simulink model "A_Robot_2_0_m_5_V22_SI"  (R2025b)
settings: Solver=VariableStepAuto  StartTime=0.0  StopTime=150  RelTol=1e-3
model workspace (MAT data in the model file):
  Km = [1; 1]
values from neighbouring files (symbols this model uses):
  kcl = kil + 50    (= 75)    [A_init_0.m]    (also in A_init_0_v2.m; A_init_1_v2.m)
  kcr = kir + 50    (= 75)    [A_init_0.m]    (also in A_init_0_v2.m; A_init_1_v2.m)
  kil = 25    [A_init_0.m]    (also in A_init_0_v2.m; A_init_1_v2.m)
  kir = 25    [A_init_0.m]    (also in A_init_0_v2.m; A_init_1_v2.m)
  kpl = 5    [A_init_0.m]    (also in A_init_0_v2.m; A_init_1_v2.m)
  kpr = 5    [A_init_0.m]    (also in A_init_0_v2.m; A_init_1_v2.m)
  theta0 = theta_0_min + (theta_0_max - theta_0_min) * rand()    [A_init_0.m]    (also in A_init_0_v2.m; A_init_1_v2.m)
  theta_gsr = theta_gsr_min + (theta_gsr_max - theta_gsr_min) * rand()    [A_init_0.m]    (also in A_init_0_v2.m; A_init_1_v2.m)
  v_rand = v_rand_0 + (v_rand_max - v_rand_0) * rand()    [A_init_0.m]    (also in A_init_0_v2.m; A_init_1_v2.m)
  x0 = x_0_min + (x_0_max - x_0_min) * rand()    [A_init_0.m]    (also in A_init_0_v2.m; A_init_1_v2.m)
  x_gsr = x_gsr_min + (x_gsr_max - x_gsr_min) * rand()    [A_init_0.m]    (also in A_init_0_v2.m; A_init_1_v2.m)
  y0 = y_0_min + (y_0_max - y_0_min) * rand()    [A_init_0.m]    (also in A_init_0_v2.m; A_init_1_v2.m)
  y_gsr = y_gsr_min + (y_gsr_max - y_gsr_min) * rand()    [A_init_0.m]    (also in A_init_0_v2.m; A_init_1_v2.m)
undefined symbols (not defined in the file or in its folder): DiscIntNeverNeededParam
libraries: simulink x15, rllib x1
(part 2 of 3)

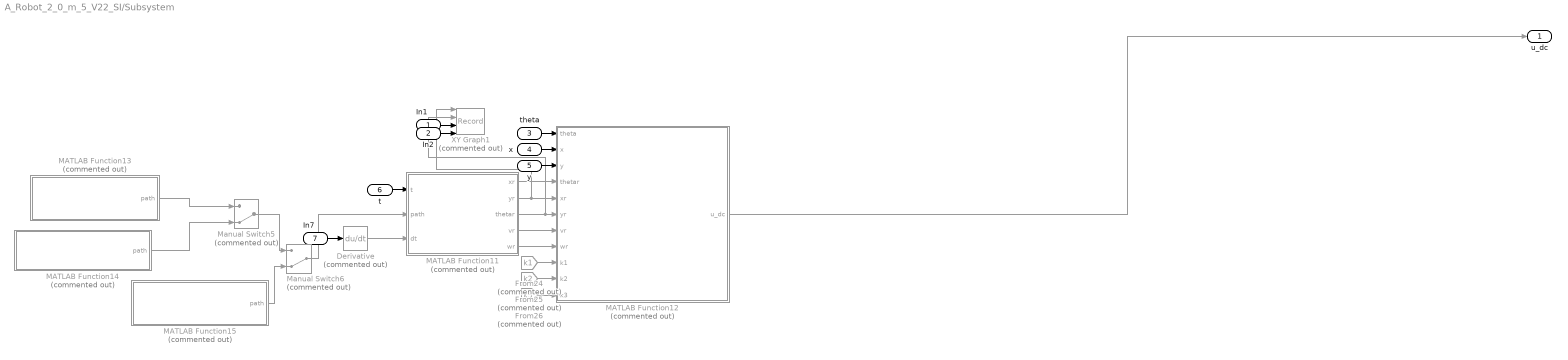
== system A_Robot_2_0_m_5_V22_SI/Subsystem ==
  In1 : Inport
  In2 : Inport  Port=2
  theta : Inport  Port=3
  x : Inport  Port=4
  y : Inport  Port=5
  t : Inport  Port=6
  In7 : Inport  Port=7
  Derivative : Derivative  Commented=on
  From24 : From  Commented=on  GotoTag=k1  TagVisibility=global
  From25 : From  Commented=on  GotoTag=k2  TagVisibility=global
  From26 : From  Commented=on  GotoTag=k3  TagVisibility=global
  MATLAB Function11 : MATLAB Function  Commented=on  TreatAsAtomicUnit=on
  MATLAB Function12 : MATLAB Function  Commented=on  TreatAsAtomicUnit=on
  MATLAB Function13 : MATLAB Function  Commented=on  TreatAsAtomicUnit=on
  MATLAB Function14 : MATLAB Function  Commented=on  TreatAsAtomicUnit=on
  MATLAB Function15 : MATLAB Function  Commented=on  TreatAsAtomicUnit=on
  Manual Switch5 : ManualSwitch  Commented=on  CurrentSetting=0
  Manual Switch6 : ManualSwitch  Commented=on  CurrentSetting=0
  XY Graph1 : Record  Commented=on  NumPorts=4.0  FileSettingsInternal="{\"entries\":[{\"content\":{\"excelSettings\":{\"content\":{},\"type\":\"Streamout.ExcelSettings\"},\"parquetSettings\":{\"content\":{},\"type\":\"Streamout.ParquetSettings\"}},\"type\":\"Streamout.FileSettingStorage\",\"uuid\":\"\"}],\"packageUris\":[\"http:\\/\\/schema.mathworks.com\\/mf0\\/streamout_blocks\\/R2020a\"],\"version\":\"1.0\"}"  FrameSettings=[0, 0, 0, 0]  Layout=[1 1]  SignalsInternal="{\"entries\":[{\"content\":{},\"type\":\"RecordBlkView.InputSignals\",\"uuid\":\"\"}],\"packageUris\":[\"http:\\/\\/schema.mathworks.com\\/mf0\\/streamout_blocks\\/R2020a\"],\"version\":\"1.0\"}"  VisualizationBindings="{\"xyplotplugin\":{\"info\":[{\"series\":[],\"subplotID\":1}]}}"  CompatibilityTag=XY
  u_dc : Outport
  wires:
  Derivative/1 -> MATLAB Function11/3(dt)
  MATLAB Function11/5(wr) -> MATLAB Function12/8(wr)
  MATLAB Function11/1(xr) -> MATLAB Function12/4(thetar)
  Manual Switch5/1 -> Manual Switch6/1
  From26/1 -> MATLAB Function12/11(k3)
  MATLAB Function14/1(path) -> Manual Switch5/2
  Manual Switch6/1 -> MATLAB Function11/2(path)
  MATLAB Function11/3(thetar) -> XY Graph1/2, MATLAB Function12/6(yr)
  MATLAB Function13/1(path) -> Manual Switch5/1
  In2/1 -> XY Graph1/4
  From25/1 -> MATLAB Function12/10(k2)
  MATLAB Function11/2(yr) -> XY Graph1/1, MATLAB Function12/5(xr)
  From24/1 -> MATLAB Function12/9(k1)
  In7/1 -> Derivative/1
  MATLAB Function15/1(path) -> Manual Switch6/2
  MATLAB Function11/4(vr) -> MATLAB Function12/7(vr)
  MATLAB Function12/1(u_dc) -> u_dc/1
  theta/1 -> MATLAB Function12/1(theta)
  x/1 -> MATLAB Function12/2(x)
  y/1 -> MATLAB Function12/3(y)
  t/1 -> MATLAB Function11/1(t)
  In1/1 -> XY Graph1/3

== system A_Robot_2_0_m_5_V22_SI/Subsystem1 ==
  + : Inport
  - : Inport  Port=2
  Demux : Demux  Outputs=2
  Demux4 : Demux  Outputs=2
  Mux7 : Mux  Inputs=2
  Sum5 : Sum  Inputs=-+|
  Sum6 : Sum  Inputs=-+|
  Out : Outport
  wires:
  Demux4/1 -> Sum5/1
  Sum5/1 -> Mux7/1
  Sum6/1 -> Mux7/2
  Demux/2 -> Sum6/2
  Demux4/2 -> Sum6/1
  Mux7/1 -> Out/1
  -/1 -> Demux4/1
  +/1 -> Demux/1
  Demux/1 -> Sum5/2

== system A_Robot_2_0_m_5_V22_SI/Subsystem10 ==
  + : Inport
  - : Inport  Port=2
  Demux : Demux  Outputs=2
  Demux4 : Demux  Outputs=2
  Mux7 : Mux  Inputs=2
  Sum5 : Sum  Inputs=-+|
  Sum6 : Sum  Inputs=-+|
  Out : Outport
  wires:
  Demux4/1 -> Sum5/1
  Sum5/1 -> Mux7/1
  Sum6/1 -> Mux7/2
  Demux/2 -> Sum6/2
  Demux4/2 -> Sum6/1
  Mux7/1 -> Out/1
  -/1 -> Demux4/1
  +/1 -> Demux/1
  Demux/1 -> Sum5/2

== system A_Robot_2_0_m_5_V22_SI/Subsystem2 ==
  + : Inport
  - : Inport  Port=2
  Demux : Demux  Outputs=2
  Demux4 : Demux  Outputs=2
  Mux7 : Mux  Inputs=2
  Sum5 : Sum  Inputs=-+|
  Sum6 : Sum  Inputs=-+|
  Out : Outport
  wires:
  Demux4/1 -> Sum5/1
  Sum5/1 -> Mux7/1
  Sum6/1 -> Mux7/2
  Demux/2 -> Sum6/2
  Demux4/2 -> Sum6/1
  Mux7/1 -> Out/1
  -/1 -> Demux4/1
  +/1 -> Demux/1
  Demux/1 -> Sum5/2

== system A_Robot_2_0_m_5_V22_SI/Subsystem3 ==
  + : Inport
  - : Inport  Port=2
  Demux : Demux  Outputs=3
  Demux4 : Demux  Outputs=3
  Mux7 : Mux  Inputs=3
  Sum1 : Sum  Inputs=-+|
  Sum5 : Sum  Inputs=-+|
  Sum6 : Sum  Inputs=-+|
  Out : Outport
  wires:
  Demux4/1 -> Sum5/1
  Sum5/1 -> Mux7/1
  Sum6/1 -> Mux7/2
  Demux/2 -> Sum6/2
  Demux4/2 -> Sum6/1
  Mux7/1 -> Out/1
  -/1 -> Demux4/1
  +/1 -> Demux/1
  Demux/1 -> Sum5/2
  Demux/3 -> Sum1/2
  Demux4/3 -> Sum1/1
  Sum1/1 -> Mux7/3

== system A_Robot_2_0_m_5_V22_SI/Subsystem4 ==
  + : Inport
  -1 : Inport  Port=2
  Demux : Demux  Outputs=3
  Demux4 : Demux  Outputs=3
  Mux7 : Mux  Inputs=3
  Sum1 : Sum  Inputs=-+|
  Sum5 : Sum  Inputs=-+|
  Sum6 : Sum  Inputs=-+|
  Out : Outport
  wires:
  Demux4/1 -> Sum5/1
  Sum5/1 -> Mux7/1
  Sum6/1 -> Mux7/2
  Demux/2 -> Sum6/2
  Demux4/2 -> Sum6/1
  Mux7/1 -> Out/1
  -1/1 -> Demux4/1
  +/1 -> Demux/1
  Demux/1 -> Sum5/2
  Demux/3 -> Sum1/2
  Demux4/3 -> Sum1/1
  Sum1/1 -> Mux7/3

== system A_Robot_2_0_m_5_V22_SI/Subsystem5 ==
  + : Inport
  - : Inport  Port=2
  Demux : Demux  Outputs=2
  Demux4 : Demux  Outputs=2
  Mux7 : Mux  Inputs=2
  Sum5 : Sum  Inputs=-+|
  Sum6 : Sum  Inputs=-+|
  Out : Outport
  wires:
  Demux4/1 -> Sum5/1
  Sum5/1 -> Mux7/1
  Sum6/1 -> Mux7/2
  Demux/2 -> Sum6/2
  Demux4/2 -> Sum6/1
  Mux7/1 -> Out/1
  -/1 -> Demux4/1
  +/1 -> Demux/1
  Demux/1 -> Sum5/2

== system A_Robot_2_0_m_5_V22_SI/Subsystem6 ==
  + : Inport
  -1 : Inport  Port=2
  Demux : Demux  Outputs=3
  Demux4 : Demux  Outputs=3
  Mux7 : Mux  Inputs=3
  Sum1 : Sum  Inputs=-+|
  Sum5 : Sum  Inputs=-+|
  Sum6 : Sum  Inputs=-+|
  Out : Outport
  wires:
  Demux4/1 -> Sum5/1
  Sum5/1 -> Mux7/1
  Sum6/1 -> Mux7/2
  Demux/2 -> Sum6/2
  Demux4/2 -> Sum6/1
  Mux7/1 -> Out/1
  -1/1 -> Demux4/1
  +/1 -> Demux/1
  Demux/1 -> Sum5/2
  Demux/3 -> Sum1/2
  Demux4/3 -> Sum1/1
  Sum1/1 -> Mux7/3

== system A_Robot_2_0_m_5_V22_SI/Subsystem7 ==
  + : Inport
  - : Inport  Port=2
  Demux : Demux  Outputs=3
  Demux4 : Demux  Outputs=3
  Mux7 : Mux  Inputs=3
  Sum1 : Sum  Inputs=-+|
  Sum5 : Sum  Inputs=-+|
  Sum6 : Sum  Inputs=-+|
  Out : Outport
  wires:
  Demux4/1 -> Sum5/1
  Sum5/1 -> Mux7/1
  Sum6/1 -> Mux7/2
  Demux/2 -> Sum6/2
  Demux4/2 -> Sum6/1
  Mux7/1 -> Out/1
  -/1 -> Demux4/1
  +/1 -> Demux/1
  Demux/1 -> Sum5/2
  Demux/3 -> Sum1/2
  Demux4/3 -> Sum1/1
  Sum1/1 -> Mux7/3

== system A_Robot_2_0_m_5_V22_SI/Subsystem8 ==
  + : Inport
  -1 : Inport  Port=2
  Demux : Demux  Outputs=3
  Demux4 : Demux  Outputs=3
  Mux7 : Mux  Inputs=3
  Sum1 : Sum  Inputs=-+|
  Sum5 : Sum  Inputs=-+|
  Sum6 : Sum  Inputs=-+|
  Out : Outport
  wires:
  Demux4/1 -> Sum5/1
  Sum5/1 -> Mux7/1
  Sum6/1 -> Mux7/2
  Demux/2 -> Sum6/2
  Demux4/2 -> Sum6/1
  Mux7/1 -> Out/1
  -1/1 -> Demux4/1
  +/1 -> Demux/1
  Demux/1 -> Sum5/2
  Demux/3 -> Sum1/2
  Demux4/3 -> Sum1/1
  Sum1/1 -> Mux7/3

== system A_Robot_2_0_m_5_V22_SI/Subsystem9 ==
  + : Inport
  - : Inport  Port=2
  Demux : Demux  Outputs=3
  Demux4 : Demux  Outputs=3
  Mux7 : Mux  Inputs=3
  Sum1 : Sum  Inputs=-+|
  Sum5 : Sum  Inputs=-+|
  Sum6 : Sum  Inputs=-+|
  Out : Outport
  wires:
  Demux4/1 -> Sum5/1
  Sum5/1 -> Mux7/1
  Sum6/1 -> Mux7/2
  Demux/2 -> Sum6/2
  Demux4/2 -> Sum6/1
  Mux7/1 -> Out/1
  -/1 -> Demux4/1
  +/1 -> Demux/1
  Demux/1 -> Sum5/2
  Demux4/3 -> Sum1/1
  Demux/3 -> Sum1/2
  Sum1/1 -> Mux7/3

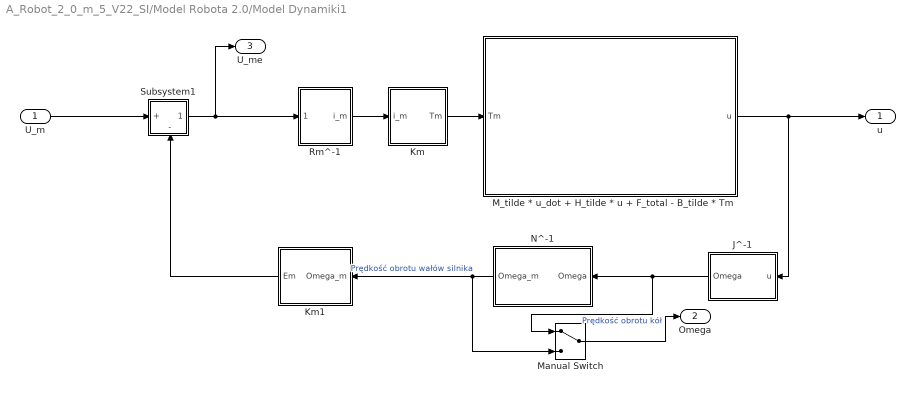
== system A_Robot_2_0_m_5_V22_SI/Model Robota 2.0/Model Dynamiki1 ==
  U_m : Inport
  J^-1 : Subsystem
  Km : Subsystem
  Km1 : Subsystem
  M_tilde * u_dot + H_tilde * u + F_total - B_tilde * Tm : Subsystem
  Manual Switch : ManualSwitch
  N^-1 : Subsystem
  Rm^-1 : Subsystem
  Subsystem1 : Subsystem
      settings: PortSchema="{\"entries\":[{\"content\":{\"sides\":[{\"content\":{\"connectorIds\":[\"In1\"]},\"type\":\"ConnectorPlacement.EquallySpacedRectSide\",\"uuid\":\"f81facd5-8dce-4a5d-a044-cb75bd1df10e\"},{\"content\":{\"connectorIds\":[\"Out1\"],\"side\":\"RIGHT\"},\"type\":\"ConnectorPlacement.EquallySpacedRectSide\",\"uuid\":\"361c4912-9b0e-4ff4-a4c3-0f951cd83b7e\"},{\"content\":{\"side\":\"TOP\"},\"type\":\"ConnectorPlacement.EquallySpacedRectSide\",\"uuid\":\"7c64f9f2-ca51-41c2-8f6b-bbae03c31185\"},{\"content\":{\"connectorIds\":[\"In2\"],\"side\":\"BOTTOM\"},\"type\":\"ConnectorPlacement.EquallySpacedRectSide\",\"uuid\":\"00962904-9a33-4c86-93c6-1e958d83cf78\"}]},\"type\":\"ConnectorPlacement.EquallySpacedConnector\",\"uuid\":\"b3c5fd64-8318-4fc9-b064-dcb9a80ffa17\"}],\"packageUris\":[\"http://schema.mathworks.com/mf0/Connector/R2020b\"],\"version\":\"1.0\"}"
  u : Outport
  Omega : Outport  Port=2
  U_me : Outport  Port=3
  wires:
  M_tilde * u_dot + H_tilde * u + F_total - B_tilde * Tm/1(u) -> J^-1/1(u), u/1
  Rm^-1/1(i_m) -> Km/1(i_m)
  Subsystem1/1(U_me) -> U_me/1, Rm^-1/1(U_me)
  N^-1/1(Omega_m) -> Manual Switch/2, Km1/1(Omega_m)  "Prędkość obrotu wałów silnika"
  J^-1/1(Omega) -> Manual Switch/1, N^-1/1(Omega)  "Prędkość obrotu kół"
  Km1/1(Em) -> Subsystem1/2(-)
  Km/1(Tm) -> M_tilde * u_dot + H_tilde * u + F_total - B_tilde * Tm/1(Tm)
  U_m/1 -> Subsystem1/1(+)
  Manual Switch/1 -> Omega/1

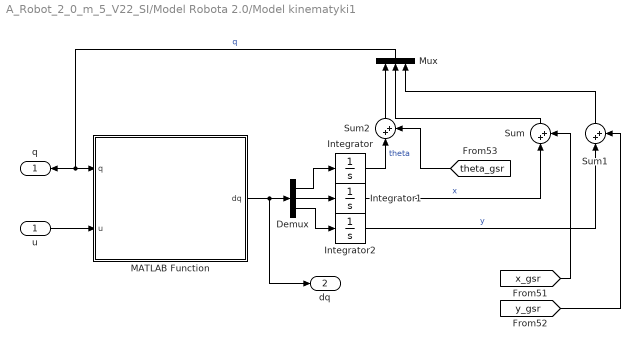
== system A_Robot_2_0_m_5_V22_SI/Model Robota 2.0/Model kinematyki1 ==
  u : Inport
  Demux : Demux  Outputs=3
  Integrator : Integrator
  Integrator1 : Integrator
  Integrator2 : Integrator
  MATLAB Function : MATLAB Function  TreatAsAtomicUnit=on
  Mux : Mux  Inputs=3
  Sum : Sum  Inputs=|++
  Sum1 : Sum  Inputs=|++
  Sum2 : Sum  Inputs=|++
  q : Outport
  dq : Outport  Port=2
  wires:
  Mux/1 -> q/1, MATLAB Function/1(q)  "q"
  Demux/1 -> Integrator/1
  Demux/3 -> Integrator2/1
  Demux/2 -> Integrator1/1
  Integrator2/1 -> Sum1/1  "y"
  MATLAB Function/1(dq) -> dq/1, Demux/1
  Integrator/1 -> Sum2/1  "theta"
  Integrator1/1 -> Sum/1  "x"
  u/1 -> MATLAB Function/2(u)
  [y_gsr] -> Sum1/2
  [x_gsr] -> Sum/2
  Sum/1 -> Mux/2
  Sum1/1 -> Mux/3
  [theta_gsr] -> Sum2/2
  Sum2/1 -> Mux/1

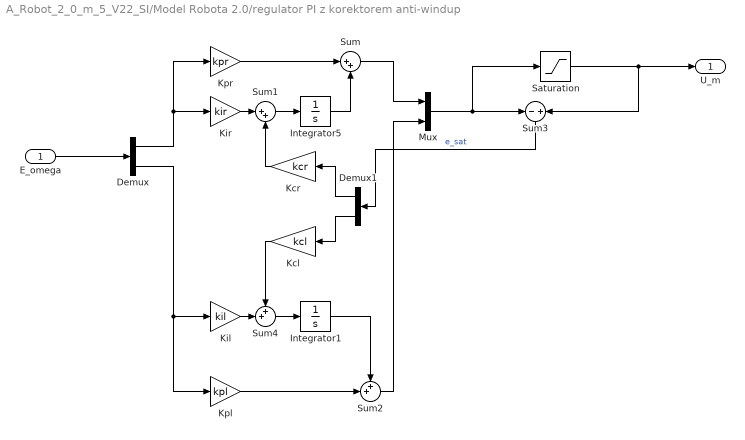
== system A_Robot_2_0_m_5_V22_SI/Model Robota 2.0/regulator PI z korektorem anti-windup ==
  E_omega : Inport
  Demux : Demux  Outputs=2
  Demux1 : Demux  Outputs=2
  Integrator1 : Integrator
  Integrator5 : Integrator
  Kcl : Gain  Gain=kcl
  Kcr : Gain  Gain=kcr
  Kil : Gain  Gain=kil
  Kir : Gain  Gain=kir
  Kpl : Gain  Gain=kpl
  Kpr : Gain  Gain=kpr
  Mux : Mux  Inputs=2
  Saturation : Saturate  UpperLimit=12  LowerLimit=-12
  Sum : Sum  Inputs=|++
  Sum1 : Sum  Inputs=|++
  Sum2 : Sum  Inputs=++|
  Sum3 : Sum  Inputs=-|+
  Sum4 : Sum  Inputs=++|
  U_m : Outport
  wires:
  Kcr/1 -> Sum1/2
  Kpr/1 -> Sum/1
  Integrator5/1 -> Sum/2
  Kir/1 -> Sum1/1
  Sum1/1 -> Integrator5/1
  Saturation/1 -> Sum3/2, U_m/1
  E_omega/1 -> Demux/1
  Demux/1 -> Kir/1, Kpr/1
  Kcl/1 -> Sum4/1
  Sum4/1 -> Integrator1/1
  Kpl/1 -> Sum2/2
  Integrator1/1 -> Sum2/1
  Kil/1 -> Sum4/2
  Demux/2 -> Kil/1, Kpl/1
  Sum3/1 -> Demux1/1  "e_sat"
  Demux1/1 -> Kcr/1
  Demux1/2 -> Kcl/1
  Sum/1 -> Mux/1
  Sum2/1 -> Mux/2
  Mux/1 -> Saturation/1, Sum3/1

== system A_Robot_2_0_m_5_V22_SI/Model Robota 2.1/Model Dynamiki1 ==
  U_m : Inport
  J^-1 : Subsystem
  Km : Subsystem
  Km1 : Subsystem
  M_tilde * u_dot + H_tilde * u + F_total - B_tilde * Tm : Subsystem
  Manual Switch : ManualSwitch
  N^-1 : Subsystem
  Rm^-1 : Subsystem
  Subsystem1 : Subsystem
      settings: PortSchema="{\"entries\":[{\"content\":{\"sides\":[{\"content\":{\"connectorIds\":[\"In1\"]},\"type\":\"ConnectorPlacement.EquallySpacedRectSide\",\"uuid\":\"f81facd5-8dce-4a5d-a044-cb75bd1df10e\"},{\"content\":{\"connectorIds\":[\"Out1\"],\"side\":\"RIGHT\"},\"type\":\"ConnectorPlacement.EquallySpacedRectSide\",\"uuid\":\"361c4912-9b0e-4ff4-a4c3-0f951cd83b7e\"},{\"content\":{\"side\":\"TOP\"},\"type\":\"ConnectorPlacement.EquallySpacedRectSide\",\"uuid\":\"7c64f9f2-ca51-41c2-8f6b-bbae03c31185\"},{\"content\":{\"connectorIds\":[\"In2\"],\"side\":\"BOTTOM\"},\"type\":\"ConnectorPlacement.EquallySpacedRectSide\",\"uuid\":\"00962904-9a33-4c86-93c6-1e958d83cf78\"}]},\"type\":\"ConnectorPlacement.EquallySpacedConnector\",\"uuid\":\"b3c5fd64-8318-4fc9-b064-dcb9a80ffa17\"}],\"packageUris\":[\"http://schema.mathworks.com/mf0/Connector/R2020b\"],\"version\":\"1.0\"}"
  u : Outport
  Omega : Outport  Port=2
  U_me : Outport  Port=3
  wires:
  M_tilde * u_dot + H_tilde * u + F_total - B_tilde * Tm/1(u) -> J^-1/1(u), u/1
  Rm^-1/1(i_m) -> Km/1(i_m)
  Subsystem1/1(U_me) -> U_me/1, Rm^-1/1(U_me)
  N^-1/1(Omega_m) -> Manual Switch/2, Km1/1(Omega_m)  "Prędkość obrotu wałów silnika"
  J^-1/1(Omega) -> Manual Switch/1, N^-1/1(Omega)  "Prędkość obrotu kół"
  Km1/1(Em) -> Subsystem1/2(-)
  Km/1(Tm) -> M_tilde * u_dot + H_tilde * u + F_total - B_tilde * Tm/1(Tm)
  U_m/1 -> Subsystem1/1(+)
  Manual Switch/1 -> Omega/1

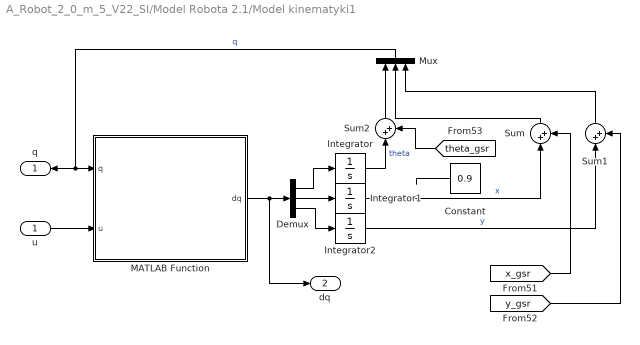
== system A_Robot_2_0_m_5_V22_SI/Model Robota 2.1/Model kinematyki1 ==
  u : Inport
  Constant : Constant  Value=0.9
  Demux : Demux  Outputs=3
  Integrator : Integrator
  Integrator1 : Integrator
  Integrator2 : Integrator
  MATLAB Function : MATLAB Function  TreatAsAtomicUnit=on
  Mux : Mux  Inputs=3
  Sum : Sum  Inputs=|++
  Sum1 : Sum  Inputs=|++
  Sum2 : Sum  Inputs=|++
  q : Outport
  dq : Outport  Port=2
  wires:
  Mux/1 -> q/1, MATLAB Function/1(q)  "q"
  Demux/1 -> Integrator/1
  Demux/3 -> Integrator2/1
  Demux/2 -> Integrator1/1
  Integrator2/1 -> Sum1/1  "y"
  MATLAB Function/1(dq) -> dq/1, Demux/1
  Integrator/1 -> Sum2/1  "theta"
  Integrator1/1 -> Sum/1  "x"
  u/1 -> MATLAB Function/2(u)
  [y_gsr] -> Sum1/2
  [x_gsr] -> Sum/2
  Sum/1 -> Mux/2
  Sum1/1 -> Mux/3
  [theta_gsr] -> Sum2/2
  Sum2/1 -> Mux/1
  Constant/1 -> ?

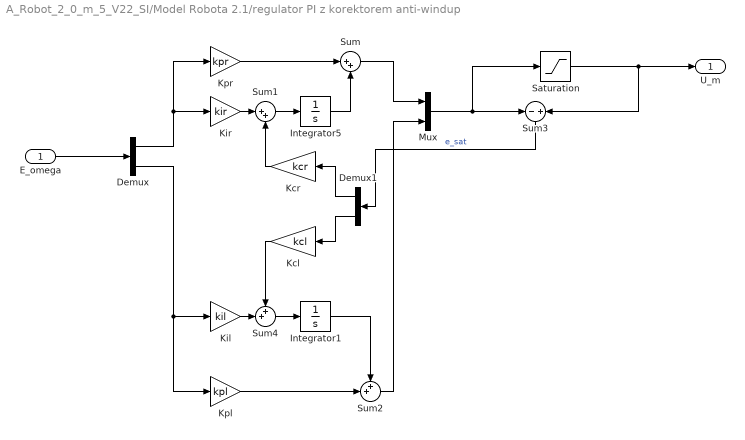
== system A_Robot_2_0_m_5_V22_SI/Model Robota 2.1/regulator PI z korektorem anti-windup ==
  E_omega : Inport
  Demux : Demux  Outputs=2
  Demux1 : Demux  Outputs=2
  Integrator1 : Integrator
  Integrator5 : Integrator
  Kcl : Gain  Gain=kcl
  Kcr : Gain  Gain=kcr
  Kil : Gain  Gain=kil
  Kir : Gain  Gain=kir
  Kpl : Gain  Gain=kpl
  Kpr : Gain  Gain=kpr
  Mux : Mux  Inputs=2
  Saturation : Saturate  UpperLimit=12  LowerLimit=-12
  Sum : Sum  Inputs=|++
  Sum1 : Sum  Inputs=|++
  Sum2 : Sum  Inputs=++|
  Sum3 : Sum  Inputs=-|+
  Sum4 : Sum  Inputs=++|
  U_m : Outport
  wires:
  Kcr/1 -> Sum1/2
  Kpr/1 -> Sum/1
  Integrator5/1 -> Sum/2
  Kir/1 -> Sum1/1
  Sum1/1 -> Integrator5/1
  Saturation/1 -> Sum3/2, U_m/1
  E_omega/1 -> Demux/1
  Demux/1 -> Kir/1, Kpr/1
  Kcl/1 -> Sum4/1
  Sum4/1 -> Integrator1/1
  Kpl/1 -> Sum2/2
  Integrator1/1 -> Sum2/1
  Kil/1 -> Sum4/2
  Demux/2 -> Kil/1, Kpl/1
  Sum3/1 -> Demux1/1  "e_sat"
  Demux1/1 -> Kcr/1
  Demux1/2 -> Kcl/1
  Sum/1 -> Mux/1
  Sum2/1 -> Mux/2
  Mux/1 -> Saturation/1, Sum3/1

== system A_Robot_2_0_m_5_V22_SI/Nagroda/Subsystem ==
  In1 : Inport
  Sqrt : Sqrt
  Square : Math  Operator=square
  Out1 : Outport
  wires:
  Square/1 -> Sqrt/1
  In1/1 -> Square/1
  Sqrt/1 -> Out1/1

== system A_Robot_2_0_m_5_V22_SI/Nagroda/Subsystem1 ==
  In1 : Inport
  Sqrt : Sqrt
  Square : Math  Operator=square
  Out1 : Outport
  wires:
  Square/1 -> Sqrt/1
  In1/1 -> Square/1
  Sqrt/1 -> Out1/1

== system A_Robot_2_0_m_5_V22_SI/Nagroda/Subsystem2 ==
  In1 : Inport
  Sqrt : Sqrt
  Square : Math  Operator=square
  Out1 : Outport
  wires:
  Square/1 -> Sqrt/1
  In1/1 -> Square/1
  Sqrt/1 -> Out1/1

== system A_Robot_2_0_m_5_V22_SI/Nagroda/Subsystem3 ==
  In1 : Inport
  Sqrt : Sqrt
  Square : Math  Operator=square
  Out1 : Outport
  wires:
  Square/1 -> Sqrt/1
  In1/1 -> Square/1
  Sqrt/1 -> Out1/1

== system A_Robot_2_0_m_5_V22_SI/Nagroda/Subsystem4 ==
  In1 : Inport
  Sqrt : Sqrt
  Square : Math  Operator=square
  Out1 : Outport
  wires:
  Square/1 -> Sqrt/1
  In1/1 -> Square/1
  Sqrt/1 -> Out1/1

== system A_Robot_2_0_m_5_V22_SI/Nagroda/Subsystem5 ==
  In1 : Inport
  Sqrt : Sqrt
  Square : Math  Operator=square
  Out1 : Outport
  wires:
  Square/1 -> Sqrt/1
  In1/1 -> Square/1
  Sqrt/1 -> Out1/1

== system A_Robot_2_0_m_5_V22_SI/Nagroda/Subsystem6 ==
  In1 : Inport
  Sqrt : Sqrt
  Square : Math  Operator=square
  Out1 : Outport
  wires:
  Square/1 -> Sqrt/1
  In1/1 -> Square/1
  Sqrt/1 -> Out1/1

== system A_Robot_2_0_m_5_V22_SI/Nagroda/Subsystem7 ==
  In1 : Inport
  Sqrt : Sqrt
  Square : Math  Operator=square
  Out1 : Outport
  wires:
  Square/1 -> Sqrt/1
  In1/1 -> Square/1
  Sqrt/1 -> Out1/1

== system A_Robot_2_0_m_5_V22_SI/Model Robota 2.0/Model Dynamiki1/J^-1 ==
  u : Inport
  MATLAB Function2 : MATLAB Function  TreatAsAtomicUnit=on
  Omega : Outport
  wires:
  MATLAB Function2/1(Omega) -> Omega/1
  [r] -> MATLAB Function2/3(r)
  [b] -> MATLAB Function2/2(b)
  u/1 -> MATLAB Function2/1(u)

== system A_Robot_2_0_m_5_V22_SI/Model Robota 2.0/Model Dynamiki1/Km ==
  i_m : Inport
  MATLAB Function2 : MATLAB Function  TreatAsAtomicUnit=on
  Tm : Outport
  wires:
  [Km] -> MATLAB Function2/2(km)
  i_m/1 -> MATLAB Function2/1(i_m)
  MATLAB Function2/1(Tm) -> Tm/1

== system A_Robot_2_0_m_5_V22_SI/Model Robota 2.0/Model Dynamiki1/Km1 ==
  Omega_m : Inport
  MATLAB Function2 : MATLAB Function  TreatAsAtomicUnit=on
  Em : Outport
  wires:
  [Km] -> MATLAB Function2/2(km)
  Omega_m/1 -> MATLAB Function2/1(Omega_m)
  MATLAB Function2/1(Em) -> Em/1

== system A_Robot_2_0_m_5_V22_SI/Model Robota 2.0/Model Dynamiki1/M_tilde * u_dot + H_tilde * u + F_total - B_tilde * Tm ==
  Tm : Inport
  B~ : Subsystem
  Demux : Demux  Outputs=2
  Fa(u) + Fr : Subsystem
  H~ : Subsystem
  Integrator : Integrator
  Integrator1 : Integrator
  Mux : Mux  Inputs=2
  M~ : Subsystem
  Subsystem1 : Subsystem
      settings: PortSchema="{\"entries\":[{\"content\":{\"sides\":[{\"content\":{\"connectorIds\":[\"In1\"]},\"type\":\"ConnectorPlacement.EquallySpacedRectSide\",\"uuid\":\"f81facd5-8dce-4a5d-a044-cb75bd1df10e\"},{\"content\":{\"connectorIds\":[\"Out1\"],\"side\":\"RIGHT\"},\"type\":\"ConnectorPlacement.EquallySpacedRectSide\",\"uuid\":\"361c4912-9b0e-4ff4-a4c3-0f951cd83b7e\"},{\"content\":{\"connectorIds\":[\"In2\"],\"side\":\"TOP\"},\"type\":\"ConnectorPlacement.EquallySpacedRectSide\",\"uuid\":\"7c64f9f2-ca51-41c2-8f6b-bbae03c31185\"},{\"content\":{\"connectorIds\":[\"In3\"],\"side\":\"BOTTOM\"},\"type\":\"ConnectorPlacement.EquallySpacedRectSide\",\"uuid\":\"00962904-9a33-4c86-93c6-1e958d83cf78\"}]},\"type\":\"ConnectorPlacement.EquallySpacedConnector\",\"uuid\":\"b3c5fd64-8318-4fc9-b064-dcb9a80ffa17\"}],\"packageUris\":[\"http://schema.mathworks.com/mf0/Connector/R2020b\"],\"version\":\"1.0\"}"
  u : Outport
  wires:
  Fa(u) + Fr/1(OUT) -> Subsystem1/2(-)
  Mux/1 -> u/1, H~/1(u), Fa(u) + Fr/1(u)  "u"
  Subsystem1/1(Out) -> M~/1(BTm)
  H~/1(OUTH) -> Subsystem1/3(-1)
  M~/1(u_d) -> Demux/1
  B~/1(BTm) -> Subsystem1/1(+)
  Tm/1 -> B~/1(Tm)
  Demux/1 -> Integrator/1
  Integrator/1 -> Mux/1
  Demux/2 -> Integrator1/1
  Integrator1/1 -> Mux/2

== system A_Robot_2_0_m_5_V22_SI/Model Robota 2.0/Model Dynamiki1/N^-1 ==
  Omega : Inport
  MATLAB Function2 : MATLAB Function  TreatAsAtomicUnit=on
  Omega_m : Outport
  wires:
  [ng] -> MATLAB Function2/2(ng)
  Omega/1 -> MATLAB Function2/1(Omega)
  MATLAB Function2/1(Omega_m) -> Omega_m/1

== system A_Robot_2_0_m_5_V22_SI/Model Robota 2.0/Model Dynamiki1/Rm^-1 ==
  U_me : Inport
  MATLAB Function : MATLAB Function  TreatAsAtomicUnit=on
  i_m : Outport
  wires:
  [R] -> MATLAB Function/2(R)
  U_me/1 -> MATLAB Function/1(U_me)
  MATLAB Function/1(i_m) -> i_m/1

== system A_Robot_2_0_m_5_V22_SI/Model Robota 2.0/Model Dynamiki1/Subsystem1 ==
  + : Inport
  - : Inport  Port=2
  Demux : Demux  Outputs=2
  Demux4 : Demux  Outputs=2
  Mux7 : Mux  Inputs=2
  Sum5 : Sum  Inputs=-+|
  Sum6 : Sum  Inputs=-+|
  U_me : Outport
  wires:
  Demux4/1 -> Sum5/1
  Sum5/1 -> Mux7/1
  Sum6/1 -> Mux7/2
  Demux/2 -> Sum6/2
  Demux4/2 -> Sum6/1
  Mux7/1 -> U_me/1
  -/1 -> Demux4/1
  +/1 -> Demux/1
  Demux/1 -> Sum5/2

== system A_Robot_2_0_m_5_V22_SI/Model Robota 2.1/Model Dynamiki1/J^-1 ==
  u : Inport
  MATLAB Function2 : MATLAB Function  TreatAsAtomicUnit=on
  Omega : Outport
  wires:
  MATLAB Function2/1(Omega) -> Omega/1
  [r] -> MATLAB Function2/3(r)
  [b] -> MATLAB Function2/2(b)
  u/1 -> MATLAB Function2/1(u)

== system A_Robot_2_0_m_5_V22_SI/Model Robota 2.1/Model Dynamiki1/Km ==
  i_m : Inport
  MATLAB Function2 : MATLAB Function  TreatAsAtomicUnit=on
  Tm : Outport
  wires:
  [Km] -> MATLAB Function2/2(km)
  i_m/1 -> MATLAB Function2/1(i_m)
  MATLAB Function2/1(Tm) -> Tm/1

== system A_Robot_2_0_m_5_V22_SI/Model Robota 2.1/Model Dynamiki1/Km1 ==
  Omega_m : Inport
  MATLAB Function2 : MATLAB Function  TreatAsAtomicUnit=on
  Em : Outport
  wires:
  [Km] -> MATLAB Function2/2(km)
  Omega_m/1 -> MATLAB Function2/1(Omega_m)
  MATLAB Function2/1(Em) -> Em/1

== system A_Robot_2_0_m_5_V22_SI/Model Robota 2.1/Model Dynamiki1/M_tilde * u_dot + H_tilde * u + F_total - B_tilde * Tm ==
  Tm : Inport
  B~ : Subsystem
  Demux : Demux  Outputs=2
  Fa(u) + Fr : Subsystem
  H~ : Subsystem
  Integrator : Integrator
  Integrator1 : Integrator
  Mux : Mux  Inputs=2
  M~ : Subsystem
  Subsystem1 : Subsystem
      settings: PortSchema="{\"entries\":[{\"content\":{\"sides\":[{\"content\":{\"connectorIds\":[\"In1\"]},\"type\":\"ConnectorPlacement.EquallySpacedRectSide\",\"uuid\":\"f81facd5-8dce-4a5d-a044-cb75bd1df10e\"},{\"content\":{\"connectorIds\":[\"Out1\"],\"side\":\"RIGHT\"},\"type\":\"ConnectorPlacement.EquallySpacedRectSide\",\"uuid\":\"361c4912-9b0e-4ff4-a4c3-0f951cd83b7e\"},{\"content\":{\"connectorIds\":[\"In2\"],\"side\":\"TOP\"},\"type\":\"ConnectorPlacement.EquallySpacedRectSide\",\"uuid\":\"7c64f9f2-ca51-41c2-8f6b-bbae03c31185\"},{\"content\":{\"connectorIds\":[\"In3\"],\"side\":\"BOTTOM\"},\"type\":\"ConnectorPlacement.EquallySpacedRectSide\",\"uuid\":\"00962904-9a33-4c86-93c6-1e958d83cf78\"}]},\"type\":\"ConnectorPlacement.EquallySpacedConnector\",\"uuid\":\"b3c5fd64-8318-4fc9-b064-dcb9a80ffa17\"}],\"packageUris\":[\"http://schema.mathworks.com/mf0/Connector/R2020b\"],\"version\":\"1.0\"}"
  u : Outport
  wires:
  Fa(u) + Fr/1(OUT) -> Subsystem1/2(-)
  Mux/1 -> u/1, H~/1(u), Fa(u) + Fr/1(u)  "u"
  Subsystem1/1(Out) -> M~/1(BTm)
  H~/1(OUTH) -> Subsystem1/3(-1)
  M~/1(u_d) -> Demux/1
  B~/1(BTm) -> Subsystem1/1(+)
  Tm/1 -> B~/1(Tm)
  Demux/1 -> Integrator/1
  Integrator/1 -> Mux/1
  Demux/2 -> Integrator1/1
  Integrator1/1 -> Mux/2

== system A_Robot_2_0_m_5_V22_SI/Model Robota 2.1/Model Dynamiki1/N^-1 ==
  Omega : Inport
  MATLAB Function2 : MATLAB Function  TreatAsAtomicUnit=on
  Omega_m : Outport
  wires:
  [ng] -> MATLAB Function2/2(ng)
  Omega/1 -> MATLAB Function2/1(Omega)
  MATLAB Function2/1(Omega_m) -> Omega_m/1

== system A_Robot_2_0_m_5_V22_SI/Model Robota 2.1/Model Dynamiki1/Rm^-1 ==
  U_me : Inport
  MATLAB Function : MATLAB Function  TreatAsAtomicUnit=on
  i_m : Outport
  wires:
  [R] -> MATLAB Function/2(R)
  U_me/1 -> MATLAB Function/1(U_me)
  MATLAB Function/1(i_m) -> i_m/1

== system A_Robot_2_0_m_5_V22_SI/Model Robota 2.1/Model Dynamiki1/Subsystem1 ==
  + : Inport
  - : Inport  Port=2
  Demux : Demux  Outputs=2
  Demux4 : Demux  Outputs=2
  Mux7 : Mux  Inputs=2
  Sum5 : Sum  Inputs=-+|
  Sum6 : Sum  Inputs=-+|
  U_me : Outport
  wires:
  Demux4/1 -> Sum5/1
  Sum5/1 -> Mux7/1
  Sum6/1 -> Mux7/2
  Demux/2 -> Sum6/2
  Demux4/2 -> Sum6/1
  Mux7/1 -> U_me/1
  -/1 -> Demux4/1
  +/1 -> Demux/1
  Demux/1 -> Sum5/2

== system A_Robot_2_0_m_5_V22_SI/Model Robota 2.0/Model Dynamiki1/M_tilde * u_dot + H_tilde * u + F_total - B_tilde * Tm/B~ ==
  Tm : Inport
  MATLAB Function8 : MATLAB Function  TreatAsAtomicUnit=on
  BTm : Outport
  wires:
  [b] -> MATLAB Function8/2(b)
  [r] -> MATLAB Function8/3(r)
  [ng] -> MATLAB Function8/4(ng)
  MATLAB Function8/1(BTm) -> BTm/1
  Tm/1 -> MATLAB Function8/1(Tm)

== system A_Robot_2_0_m_5_V22_SI/Model Robota 2.0/Model Dynamiki1/M_tilde * u_dot + H_tilde * u + F_total - B_tilde * Tm/Fa(u) + Fr ==
  u : Inport
  Demux : Demux  Outputs=2
  MATLAB Function7 : MATLAB Function  TreatAsAtomicUnit=on
  OUT : Outport
  wires:
  u/1 -> Demux/1
  [r] -> MATLAB Function7/3(r)
  [m] -> MATLAB Function7/4(m)
  [b] -> MATLAB Function7/5(b)
  MATLAB Function7/1(OUT) -> OUT/1
  Demux/1 -> MATLAB Function7/1(omega)
  Demux/2 -> MATLAB Function7/2(v)

== system A_Robot_2_0_m_5_V22_SI/Model Robota 2.0/Model Dynamiki1/M_tilde * u_dot + H_tilde * u + F_total - B_tilde * Tm/H~ ==
  u : Inport
  MATLAB Function6 : MATLAB Function  TreatAsAtomicUnit=on
  OUTH : Outport
  wires:
  [r] -> MATLAB Function6/5(r)
  [b] -> MATLAB Function6/6(b)
  [xi_m] -> MATLAB Function6/3(xi_m)
  MATLAB Function6/1(OUTH) -> OUTH/1
  [xi] -> MATLAB Function6/2(xi)
  [ng] -> MATLAB Function6/4(ng)
  u/1 -> MATLAB Function6/1(u)

== system A_Robot_2_0_m_5_V22_SI/Model Robota 2.0/Model Dynamiki1/M_tilde * u_dot + H_tilde * u + F_total - B_tilde * Tm/M~ ==
  BTm : Inport
  MATLAB Function : MATLAB Function  TreatAsAtomicUnit=on
  MATLAB Function2 : MATLAB Function  TreatAsAtomicUnit=on
  u_d : Outport
  wires:
  [r] -> MATLAB Function/6(r)
  [In] -> MATLAB Function/4(Im)
  [m] -> MATLAB Function2/1(m)
  [m] -> MATLAB Function/5(m)
  [b] -> MATLAB Function/7(b)
  MATLAB Function2/1(Ic) -> MATLAB Function/2(Ic)
  [ng] -> MATLAB Function/8(ng)
  [b] -> MATLAB Function2/2(b)
  [Ik] -> MATLAB Function/3(Ik)
  BTm/1 -> MATLAB Function/1(BTm)
  MATLAB Function/1(u_d) -> u_d/1

== system A_Robot_2_0_m_5_V22_SI/Model Robota 2.0/Model Dynamiki1/M_tilde * u_dot + H_tilde * u + F_total - B_tilde * Tm/Subsystem1 ==
  + : Inport
  - : Inport  Port=2
  -1 : Inport  Port=3
  Demux : Demux  Outputs=2
  Demux1 : Demux  Outputs=2
  Demux4 : Demux  Outputs=2
  Mux7 : Mux  Inputs=2
  Sum1 : Sum  Inputs=-+-|
  Sum5 : Sum  Inputs=-+-|
  Out : Outport
  wires:
  Demux4/1 -> Sum5/1
  Sum5/1 -> Mux7/1
  Sum1/1 -> Mux7/2
  Demux/2 -> Sum1/2
  Demux4/2 -> Sum1/1
  Mux7/1 -> Out/1
  -/1 -> Demux4/1
  +/1 -> Demux/1
  Demux/1 -> Sum5/2
  -1/1 -> Demux1/1
  Demux1/1 -> Sum5/3
  Demux1/2 -> Sum1/3

== system A_Robot_2_0_m_5_V22_SI/Model Robota 2.1/Model Dynamiki1/M_tilde * u_dot + H_tilde * u + F_total - B_tilde * Tm/B~ ==
  Tm : Inport
  MATLAB Function8 : MATLAB Function  TreatAsAtomicUnit=on
  BTm : Outport
  wires:
  [b] -> MATLAB Function8/2(b)
  [r] -> MATLAB Function8/3(r)
  [ng] -> MATLAB Function8/4(ng)
  MATLAB Function8/1(BTm) -> BTm/1
  Tm/1 -> MATLAB Function8/1(Tm)

== system A_Robot_2_0_m_5_V22_SI/Model Robota 2.1/Model Dynamiki1/M_tilde * u_dot + H_tilde * u + F_total - B_tilde * Tm/Fa(u) + Fr ==
  u : Inport
  Demux : Demux  Outputs=2
  MATLAB Function7 : MATLAB Function  TreatAsAtomicUnit=on
  OUT : Outport
  wires:
  u/1 -> Demux/1
  [r] -> MATLAB Function7/3(r)
  [m] -> MATLAB Function7/4(m)
  [b] -> MATLAB Function7/5(b)
  MATLAB Function7/1(OUT) -> OUT/1
  Demux/1 -> MATLAB Function7/1(omega)
  Demux/2 -> MATLAB Function7/2(v)

== system A_Robot_2_0_m_5_V22_SI/Model Robota 2.1/Model Dynamiki1/M_tilde * u_dot + H_tilde * u + F_total - B_tilde * Tm/H~ ==
  u : Inport
  MATLAB Function6 : MATLAB Function  TreatAsAtomicUnit=on
  OUTH : Outport
  wires:
  [r] -> MATLAB Function6/5(r)
  [b] -> MATLAB Function6/6(b)
  [xi_m] -> MATLAB Function6/3(xi_m)
  MATLAB Function6/1(OUTH) -> OUTH/1
  [xi] -> MATLAB Function6/2(xi)
  [ng] -> MATLAB Function6/4(ng)
  u/1 -> MATLAB Function6/1(u)

== system A_Robot_2_0_m_5_V22_SI/Model Robota 2.1/Model Dynamiki1/M_tilde * u_dot + H_tilde * u + F_total - B_tilde * Tm/M~ ==
  BTm : Inport
  MATLAB Function : MATLAB Function  TreatAsAtomicUnit=on
  MATLAB Function2 : MATLAB Function  TreatAsAtomicUnit=on
  u_d : Outport
  wires:
  [r] -> MATLAB Function/6(r)
  [In] -> MATLAB Function/4(Im)
  [m] -> MATLAB Function2/1(m)
  [m] -> MATLAB Function/5(m)
  [b] -> MATLAB Function/7(b)
  MATLAB Function2/1(Ic) -> MATLAB Function/2(Ic)
  [ng] -> MATLAB Function/8(ng)
  [b] -> MATLAB Function2/2(b)
  [Ik] -> MATLAB Function/3(Ik)
  BTm/1 -> MATLAB Function/1(BTm)
  MATLAB Function/1(u_d) -> u_d/1

== system A_Robot_2_0_m_5_V22_SI/Model Robota 2.1/Model Dynamiki1/M_tilde * u_dot + H_tilde * u + F_total - B_tilde * Tm/Subsystem1 ==
  + : Inport
  - : Inport  Port=2
  -1 : Inport  Port=3
  Demux : Demux  Outputs=2
  Demux1 : Demux  Outputs=2
  Demux4 : Demux  Outputs=2
  Mux7 : Mux  Inputs=2
  Sum1 : Sum  Inputs=-+-|
  Sum5 : Sum  Inputs=-+-|
  Out : Outport
  wires:
  Demux4/1 -> Sum5/1
  Sum5/1 -> Mux7/1
  Sum1/1 -> Mux7/2
  Demux/2 -> Sum1/2
  Demux4/2 -> Sum1/1
  Mux7/1 -> Out/1
  -/1 -> Demux4/1
  +/1 -> Demux/1
  Demux/1 -> Sum5/2
  -1/1 -> Demux1/1
  Demux1/1 -> Sum5/3
  Demux1/2 -> Sum1/3

== matlab function A_Robot_2_0_m_5_V22_SI/J^-1/MATLAB Function8 ==
  data: u_dc input; Omega_dc output; r input; b input
function Omega_dc  = konwersja(u_dc, r, b)
    % Przekształcenie prędkości platformy na prędkości kół
    
    
    % Macierz J^{-1} przekształcająca u -> Omega
J_1 = [b/r, 1/r;
      -b/r, 1/r];
    % Obliczenie prędkości kątowych kół
    Omega_dc = J_1 * u_dc;


end

== matlab function A_Robot_2_0_m_5_V22_SI/MATLAB Function9 ==
  data: v_rand input; t input; theta_d_out output; dx_d output; dy_d output; theta_d input; v_d output
function [theta_d_out, dx_d, dy_d, v_d] = GSR(v_rand, t, theta_d)
    v_d = v_rand;
    dx_d = v_d * cos(theta_d);
    dy_d = v_d * sin(theta_d);
    theta_d_out = theta_d;

end

== matlab function A_Robot_2_0_m_5_V22_SI/MATLAB Function10 ==
  data: t input; dtheta_d output
function dtheta_d = obl_theta(t)
    omega_d =0.0;
    dtheta_d = omega_d;

end

== matlab function A_Robot_2_0_m_5_V22_SI/Subsystem/MATLAB Function11 ==
  data: t input; xr output; path input; dt input; yr output; thetar output; vr output; wr output
function [xr, yr, thetar, vr, wr] = GSR_from_path(t, path, dt)
    % Generator sygnałów referencyjnych ze ścieżki (dowolnego wykresu)
    % path: Nx2 macierz punktów [x y]
    % t: czas
    % dt: krok czasowy symulacji

    % Przejście po punktach w tempie odpowiadającym dt
    i = floor(t / dt) + 1;
    i_next = min(i + 1, size(path, 1));
    
    % Bieżący i kolejny punkt
    p1 = path(i, :);
    p2 = path(i_next, :);

    % Pozycja referencyjna
    xr = p1(1);
    yr = p1(2);

    % Różnice
    dx = p2(1) - p1(1);
    dy = p2(2) - p1(2);

    % Prędkość liniowa (różniczkowanie)
    vr = sqrt(dx^2 + dy^2) / dt;

    % Orientacja (kierunek trajektorii)
    thetar = atan2(dy, dx);

    % Przybliżona prędkość kątowa (zmiana kierunku)
    if i < size(path, 1) - 1
        p3 = path(min(i + 2, size(path, 1)), :);
        dtheta1 = atan2(p2(2) - p1(2), p2(1) - p1(1));
        dtheta2 = atan2(p3(2) - p2(2), p3(1) - p2(1));
        dtheta = wrapToPi(dtheta2 - dtheta1);
        wr = dtheta / dt;
    else
        wr = 0;
    end
end

== matlab function A_Robot_2_0_m_5_V22_SI/Subsystem/MATLAB Function12 ==
  data: theta input; x input; y input; thetar input; xr input; yr input; u_dc output; vr input; wr input; k1 input; k2 input; k3 input
function u_dc  = ASP(theta, x, y, thetar, xr, yr, vr, wr, k1, k2, k3)


    % Obliczenie błędów pozycji w lokalnym układzie robota
    dx = xr - x;
    dy = yr - y;
    dtheta = wrapToPi(thetar - theta);

    % Przekształcenie błędów pozycji do układu robota
    e1 =  cos(theta) * dx + sin(theta) * dy;
    e2 = -sin(theta) * dx + cos(theta) * dy;
    e3 = dtheta;

    % Kinematyczna reguła sterowania
    v_c     = vr * cos(e3) + k1 * e1;
    omega_c = wr + k2 * vr * e2 + k3 * vr * sin(e3);

    u_dc=[omega_c;v_c];
end

== matlab function A_Robot_2_0_m_5_V22_SI/Subsystem/MATLAB Function13 ==
  data: path output
function path = generate_path_rectangle()
    % Prosta ścieżka prostokątna z 4 narożnikami

    % Wierzchołki prostokąta
    p = [0 0;
         1 0;
         1 1;
         0 1;
         0 0];

    % Interpolacja — gęstość punktów między wierzchołkami
    N = 20;  % liczba punktów na bok

    path = [];

    for i = 1:size(p,1)-1
        x = linspace(p(i,1), p(i+1,1), N)';
        y = linspace(p(i,2), p(i+1,2), N)';
        path = [path; [x y]];
    end
end

== matlab function A_Robot_2_0_m_5_V22_SI/Subsystem/MATLAB Function14 ==
  data: path output
function path = generate_path_sinusoidal()
    % Ścieżka sinusoidalna wzdłuż osi X

    x = linspace(0, 5, 200)';
    y = 0.5 * sin(2 * pi * x / 5);

    path = [x y];
end

== matlab function A_Robot_2_0_m_5_V22_SI/Subsystem/MATLAB Function15 ==
  data: path output
function path = generate_path_circle()
    % Okrąg o promieniu R

    R = 1.0;
    N = 200;
    theta = linspace(0, 2*pi, N)';

    x = R * cos(theta);
    y = R * sin(theta);

    path = [x y];
end

== matlab function A_Robot_2_0_m_5_V22_SI/Model kinematyki1/MATLAB Function ==
  data: q input; u input; dq output
function dq = kinematyka(q, u)
% Wejście:
%   q - wektor stanu [theta; x; y]
%   u - wektor sterowania [omega; v] (prędkość kątowa i liniowa)
% Wyjście:
%   dq - pochodne stanu [dtheta; dx; dy] uwzględniające ograniczenie Pfaffa
dq=[0;0;0];
% Rozpakowanie wektora stanu
theta = q(1);  % Kąt orientacji robota
x = q(2);      % Pozycja x
y = q(3);      % Pozycja y

% Macierz kinematyki G(q)
Gq = [1,  0;
      0, cos(theta);
      0, sin(theta)];

% Wstępna pochodna stanu
dq = Gq * u;

end

== matlab function A_Robot_2_0_m_5_V22_SI/Model Robota 2.1/Model Dynamiki1/Km1/MATLAB Function2 ==
  data: Omega_m input; km input; Em output
function Em=Km(Omega_m,km)
% Oblicza momenty napędowe Tm na podstawie prądów silników i_m
%
% Wejście:
%   i_m  – wektor prądów silników [i_mP; i_mL] (A)
%   km   – stała maszynowa silnika [N·m/A]
%
% Wyjście:
%   Tm   – wektor momentów napędowych [Tm_P; Tm_L] (N·m)

% Stała maszynowa jako macierz diagonalna
Km = km * eye(2);

% Obliczenie momentów napędowych
Em = Km * Omega_m;

end

== matlab function A_Robot_2_0_m_5_V22_SI/Model Robota 2.0/Model Dynamiki1/M_tilde * u_dot + H_tilde * u + F_total - B_tilde * Tm/M~/MATLAB Function2 ==
  data: m input; Ic output; b input
function Ic = moment(m,b)

B=b;

Ic = m*(B^2+B^2)/12;

== matlab function A_Robot_2_0_m_5_V22_SI/Model Robota 2.1/Model Dynamiki1/M_tilde * u_dot + H_tilde * u + F_total - B_tilde * Tm/B~/MATLAB Function8 ==
  data: Tm input; b input; BTm output; r input; ng input
function BTm = B_tilde(Tm, b, r, ng)
    % Oblicza macierz B~ zgodnie ze wzorem (2.65)
    %
    % b  – połowa rozstawu kół [m]
    % r  – promień koła [m]
    % ng – przełożenie przekładni [-]

    wsp = 1 / (r * ng);

    B_tilde = [ b * wsp, -b * wsp;
                wsp,     wsp ];

    BTm = B_tilde * Tm;
end

== matlab function A_Robot_2_0_m_5_V22_SI/Model Robota 2.1/Model Dynamiki1/M_tilde * u_dot + H_tilde * u + F_total - B_tilde * Tm/Fa(u) + Fr/MATLAB Function7 ==
  data: omega input; v input; OUT output; r input; m input; b input
function OUT = F(omega, v, r, m, b)
    % Oblicza łączną siłę oporu powietrza i toczenia kół:
    % F_total = Fa(u) + Fr(omegaP, omegaL)
    %
    % Wejścia:
    % v       – prędkość liniowa platformy [m/s]
    % omegaP  – prędkość kątowa prawego koła [rad/s]
    % omegaL  – prędkość kątowa lewego koła [rad/s]
    % param          Daw, Dav, Cr, nu, g,
g   = 9.81;     % przyspieszenie ziemskie [m/s²]
Cr  = 5e-4;     % współczynnik oporu toczenia [-]
Daw = 5e-4;     % opór aerodynamiczny obrotowy [kg·m²/s]
Dav = 5e-3;      % opór aerodynamiczny liniowy [kg/m]
nu  = 10;        % współczynnik stromości funkcji tanh [-]


    % --- Prędkości kół ---
    omegaP = v + b * omega;
    omegaL = v - b * omega;

    % --- Fa: opór powietrza ---
    Na = Daw * abs(omega) * omega;   
    Fa = Dav * abs(v) * v;

    F_a = [Na; Fa];  % zgodnie ze wzorem (2.41)

    % --- Fr: opór toczenia ---
    rwP = r * omegaP;
    rwL = r * omegaL;

    Nr = (b/2) * m * g * Cr * (tanh(nu * rwP) - tanh(nu * rwL));
    Fr = (1/2) * m * g * Cr * (tanh(nu * rwP) + tanh(nu * rwL));

    F_r = [Nr; Fr];  % zgodnie ze wzorem (2.46)

    % --- Suma sił oporu ---
    F_total = F_a + F_r;

    OUT = F_total;


end

== matlab function A_Robot_2_0_m_5_V22_SI/MATLAB Function1 ==
  data: t input; dtheta_d output
function dtheta_d = obl_theta(t)
    % Figury Lissajousa: x = cos(t), y = sin(2t)
    dx = cos(t);
    dy = sin(2*t);

    ddx = -sin(t);
    ddy = 2 * cos(2*t);

    dtheta_d = (ddy * dx - ddx * dy) / (dx^2 + dy^2);
end

== matlab function A_Robot_2_0_m_5_V22_SI/Model Robota 2.1/Model Dynamiki1/M_tilde * u_dot + H_tilde * u + F_total - B_tilde * Tm/H~/MATLAB Function6 ==
  data: u input; xi input; OUTH output; xi_m input; ng input; r input; b input
function OUTH = H_tilde(u, xi, xi_m, ng, r, b)
    % Oblicza macierz H~ według wzoru (2.64), z pełnym rozwinięciem składników
    %
    % xi     – tłumienie w łożyskach kół [N·m·s]
    % xi_m   – tłumienie w łożyskach silników [N·m·s]
    % ng     – przełożenie przekładni [-]
    % r      – promień koła [m]
    % b      – połowa rozstawu kół [m]

    % Składowe macierzy
    H11 = (2 * b^2 / r^2) * xi ...
         + (2 * b^2 / (r^2 * ng^2)) * xi_m;

    H12 = 0;

    H21 = 0;

    H22 = (2 / r^2) * xi ...
         + (2 / (r^2 * ng^2)) * xi_m;

    % Macierz wynikowa
    H_tilde = [H11, H12;
               H21, H22];

    OUTH = H_tilde * u;
end

== matlab function A_Robot_2_0_m_5_V22_SI/Model Robota 2.0/Model Dynamiki1/M_tilde * u_dot + H_tilde * u + F_total - B_tilde * Tm/M~/MATLAB Function ==
  data: BTm input; Ic input; u_d output; Ik input; Im input; m input; r input; b input; ng input
function u_d = M_tilde(BTm, Ic, Ik, Im, m, r, b, ng)
    % Funkcja oblicza macierz M~ (M_tilde) zgodnie ze wzorem (2.63)
    %
    % Ic  – moment bezwładności platformy wokół osi obrotu
    % Ik  – moment bezwładności kół
    % Im  – moment bezwładności silników
    % m   – masa platformy
    % r   – promień koła
    % b   – połowa rozstawu osi
    % ng  – przełożenie przekładni

M_tilde1 = [Ic + (((2 * b^2) / r^2) * Ik) + ((2 * b^2) / (r^2 * ng^2)) * Im, 0;
               0, m + (((2) / r^2) * Ik) + ((2) / (r^2 * ng^2)) * Im];
M_tilde = inv(M_tilde1);
u_d = M_tilde * BTm;
end

== matlab function A_Robot_2_0_m_5_V22_SI/Model Robota 2.0/Model Dynamiki1/M_tilde * u_dot + H_tilde * u + F_total - B_tilde * Tm/H~/MATLAB Function6 ==
  data: u input; xi input; OUTH output; xi_m input; ng input; r input; b input
function OUTH = H_tilde(u, xi, xi_m, ng, r, b)
    % Oblicza macierz H~ według wzoru (2.64), z pełnym rozwinięciem składników
    %
    % xi     – tłumienie w łożyskach kół [N·m·s]
    % xi_m   – tłumienie w łożyskach silników [N·m·s]
    % ng     – przełożenie przekładni [-]
    % r      – promień koła [m]
    % b      – połowa rozstawu kół [m]

    % Składowe macierzy
    H11 = (2 * b^2 / r^2) * xi ...
         + (2 * b^2 / (r^2 * ng^2)) * xi_m;

    H12 = 0;

    H21 = 0;

    H22 = (2 / r^2) * xi ...
         + (2 / (r^2 * ng^2)) * xi_m;

    % Macierz wynikowa
    H_tilde = [H11, H12;
               H21, H22];

    OUTH = H_tilde * u;
end

== matlab function A_Robot_2_0_m_5_V22_SI/Model Robota 2.0/Model Dynamiki1/M_tilde * u_dot + H_tilde * u + F_total - B_tilde * Tm/Fa(u) + Fr/MATLAB Function7 ==
  data: omega input; v input; OUT output; r input; m input; b input
function OUT = F(omega, v, r, m, b)
    % Oblicza łączną siłę oporu powietrza i toczenia kół:
    % F_total = Fa(u) + Fr(omegaP, omegaL)
    %
    % Wejścia:
    % v       – prędkość liniowa platformy [m/s]
    % omegaP  – prędkość kątowa prawego koła [rad/s]
    % omegaL  – prędkość kątowa lewego koła [rad/s]
    % param          Daw, Dav, Cr, nu, g,
g   = 9.81;     % przyspieszenie ziemskie [m/s²]
Cr  = 5e-4;     % współczynnik oporu toczenia [-]
Daw = 5e-4;     % opór aerodynamiczny obrotowy [kg·m²/s]
Dav = 5e-3;      % opór aerodynamiczny liniowy [kg/m]
nu  = 10;        % współczynnik stromości funkcji tanh [-]


    % --- Prędkości kół ---
    omegaP = v + b * omega;
    omegaL = v - b * omega;

    % --- Fa: opór powietrza ---
    Na = Daw * abs(omega) * omega;   
    Fa = Dav * abs(v) * v;

    F_a = [Na; Fa];  % zgodnie ze wzorem (2.41)

    % --- Fr: opór toczenia ---
    rwP = r * omegaP;
    rwL = r * omegaL;

    Nr = (b/2) * m * g * Cr * (tanh(nu * rwP) - tanh(nu * rwL));
    Fr = (1/2) * m * g * Cr * (tanh(nu * rwP) + tanh(nu * rwL));

    F_r = [Nr; Fr];  % zgodnie ze wzorem (2.46)

    % --- Suma sił oporu ---
    F_total = F_a + F_r;

    OUT = F_total;


end

== matlab function A_Robot_2_0_m_5_V22_SI/Model Robota 2.0/Model kinematyki1/MATLAB Function ==
  data: q input; u input; dq output
function dq = kinematyka(q, u)
% Wejście:
%   q - wektor stanu [theta; x; y]
%   u - wektor sterowania [omega; v] (prędkość kątowa i liniowa)
% Wyjście:
%   dq - pochodne stanu [dtheta; dx; dy] uwzględniające ograniczenie Pfaffa
dq=[0;0;0];
% Rozpakowanie wektora stanu
theta = q(1);  % Kąt orientacji robota
x = q(2);      % Pozycja x
y = q(3);      % Pozycja y

% Macierz kinematyki G(q)
Gq = [1,  0;
      0, cos(theta);
      0, sin(theta)];

% Wstępna pochodna stanu
dq = Gq * u;

end

== matlab function A_Robot_2_0_m_5_V22_SI/Model Robota 2.0/Model Dynamiki1/M_tilde * u_dot + H_tilde * u + F_total - B_tilde * Tm/B~/MATLAB Function8 ==
  data: Tm input; b input; BTm output; r input; ng input
function BTm = B_tilde(Tm, b, r, ng)
    % Oblicza macierz B~ zgodnie ze wzorem (2.65)
    %
    % b  – połowa rozstawu kół [m]
    % r  – promień koła [m]
    % ng – przełożenie przekładni [-]

    wsp = 1 / (r * ng);

    B_tilde = [ b * wsp, -b * wsp;
                wsp,     wsp ];

    BTm = B_tilde * Tm;
end

== matlab function A_Robot_2_0_m_5_V22_SI/Model Robota 2.0/Model Dynamiki1/Km/MATLAB Function2 ==
  data: i_m input; Tm output; km input
function Tm = Km(i_m, km)
% Oblicza momenty napędowe Tm na podstawie prądów silników i_m
%
% Wejście:
%   i_m  – wektor prądów silników [i_mP; i_mL] (A)
%   km   – stała maszynowa silnika [N·m/A]
%
% Wyjście:
%   Tm   – wektor momentów napędowych [Tm_P; Tm_L] (N·m)

% Stała maszynowa jako macierz diagonalna
Km = km * eye(2);

% Obliczenie momentów napędowych
Tm = Km * i_m;

end

== matlab function A_Robot_2_0_m_5_V22_SI/MATLAB Function ==
  data: t input; dx_r output; dy_r output; theta_r output; v_r output; omega_r output
function [dx_r, dy_r, theta_r, v_r, omega_r] = GSR_trajektoria(t)
    % Parametry trajektorii ósemkowej
    A = 0.5; B = 0.25; w = 0.1;

 % Prędkości (pochodne pozycji)
    dx_r = A * w * cos(w * t);
    dy_r = B * w * (cos(2*w*t) - sin(2*w*t));

    % Przyspieszenia (pochodne prędkości)
    ddx = -A * w^2 * sin(w * t);
    ddy = -2 * B * w^2 * sin(2*w*t);

    % Prędkość liniowa
    v_r = sqrt(dx_r^2 + dy_r^2);

    % Kąt orientacji
    theta_r = atan2(dy_r, dx_r);

    % Prędkość kątowa (pochodna theta)
    omega_r = (ddy * dx_r - ddx * dy_r) / (dx_r^2 + dy_r^2);
end

== matlab function A_Robot_2_0_m_5_V22_SI/Model Robota 2.0/Model Dynamiki1/Rm^-1/MATLAB Function ==
  data: U_me input; i_m output; R input
function i_m = R_m1(U_me, R)
% Oblicza wektor prądów silników i_m = R^{-1} * (U_m - E_m)
%
% Wejścia:
%   U_m – wektor napięć sterujących [U_mP; U_mL] (V)
%   R   – rezystancja uzwojeń (skalar) lub macierz 2x2
R = eye(2) * R;

i_m = inv(R) * U_me;  % bardziej wydajna wersja niż inv(R) * (U - E)

end

== matlab function A_Robot_2_0_m_5_V22_SI/Model Robota 2.0/Model Dynamiki1/J^-1/MATLAB Function2 ==
  data: u input; Omega output; b input; r input
function Omega = predkosc_kotawa_kol(u, b, r)
% Oblicza prędkości kątowe kół napędowych Omega = [omega_P; omega_L]
% na podstawie wektora prędkości platformy u = [omega; v]
%
% Wejście:
%   u   - wektor prędkości platformy [omega; v] (rad/s, m/s)
%   b   - połowa rozstawu kół (odległość od osi do koła) [m]
%   r   - promień koła [m]
%
% Wyjście:
%   Omega - wektor prędkości kół [omega_P; omega_L] (rad/s)

% Macierz J^{-1} przekształcająca u -> Omega
J_1 = [b/r,1/r;
      -b/r,1/r];

% Obliczenie prędkości kątowych kół
Omega = J_1 * u;

end

== matlab function A_Robot_2_0_m_5_V22_SI/Model Robota 2.0/Model Dynamiki1/N^-1/MATLAB Function2 ==
  data: Omega input; Omega_m output; ng input
function Omega_m = predkosc_kotawa_walow(Omega, ng)
% Oblicza prędkości kątowe wałów silników Omega_m
% na podstawie prędkości kół napędowych Omega = [omega_P; omega_L]
%
% Wejście:
%   Omega - wektor prędkości kół [omega_P; omega_L] (rad/s)
%   ng    - przełożenie przekładni redukcyjnej (ng < 1) [-]
%
% Wyjście:
%   Omega_m - prędkości kątowe wałów silników [omega_mP; omega_mL] (rad/s)

% Macierz odwrotności przełożenia
Ninv = (1/ng) * eye(2);

% Obliczenie prędkości wałów silników
Omega_m = Ninv * Omega;

end

== matlab function A_Robot_2_0_m_5_V22_SI/Model Robota 2.0/Model Dynamiki1/Km1/MATLAB Function2 ==
  data: Omega_m input; km input; Em output
function Em=Km(Omega_m,km)
% Oblicza momenty napędowe Tm na podstawie prądów silników i_m
%
% Wejście:
%   i_m  – wektor prądów silników [i_mP; i_mL] (A)
%   km   – stała maszynowa silnika [N·m/A]
%
% Wyjście:
%   Tm   – wektor momentów napędowych [Tm_P; Tm_L] (N·m)

% Stała maszynowa jako macierz diagonalna
Km = km * eye(2);

% Obliczenie momentów napędowych
Em = Km * Omega_m;

end

== matlab function A_Robot_2_0_m_5_V22_SI/Model Robota 2.1/Model Dynamiki1/M_tilde * u_dot + H_tilde * u + F_total - B_tilde * Tm/M~/MATLAB Function ==
  data: BTm input; Ic input; u_d output; Ik input; Im input; m input; r input; b input; ng input
function u_d = M_tilde(BTm, Ic, Ik, Im, m, r, b, ng)
    % Funkcja oblicza macierz M~ (M_tilde) zgodnie ze wzorem (2.63)
    %
    % Ic  – moment bezwładności platformy wokół osi obrotu
    % Ik  – moment bezwładności kół
    % Im  – moment bezwładności silników
    % m   – masa platformy
    % r   – promień koła
    % b   – połowa rozstawu osi
    % ng  – przełożenie przekładni

M_tilde1 = [Ic + (((2 * b^2) / r^2) * Ik) + ((2 * b^2) / (r^2 * ng^2)) * Im, 0;
               0, m + (((2) / r^2) * Ik) + ((2) / (r^2 * ng^2)) * Im];
M_tilde = inv(M_tilde1);
u_d = M_tilde * BTm;
end

== matlab function A_Robot_2_0_m_5_V22_SI/Model Robota 2.1/Model Dynamiki1/M_tilde * u_dot + H_tilde * u + F_total - B_tilde * Tm/M~/MATLAB Function2 ==
  data: m input; Ic output; b input
function Ic = moment(m,b)

B=b;

Ic = m*(B^2+B^2)/12;

== matlab function A_Robot_2_0_m_5_V22_SI/Model Robota 2.1/Model Dynamiki1/N^-1/MATLAB Function2 ==
  data: Omega input; Omega_m output; ng input
function Omega_m = predkosc_kotawa_walow(Omega, ng)
% Oblicza prędkości kątowe wałów silników Omega_m
% na podstawie prędkości kół napędowych Omega = [omega_P; omega_L]
%
% Wejście:
%   Omega - wektor prędkości kół [omega_P; omega_L] (rad/s)
%   ng    - przełożenie przekładni redukcyjnej (ng < 1) [-]
%
% Wyjście:
%   Omega_m - prędkości kątowe wałów silników [omega_mP; omega_mL] (rad/s)

% Macierz odwrotności przełożenia
Ninv = (1/ng) * eye(2);

% Obliczenie prędkości wałów silników
Omega_m = Ninv * Omega;

end

== matlab function A_Robot_2_0_m_5_V22_SI/Model Robota 2.1/Model Dynamiki1/Rm^-1/MATLAB Function ==
  data: U_me input; i_m output; R input
function i_m = R_m1(U_me, R)
% Oblicza wektor prądów silników i_m = R^{-1} * (U_m - E_m)
%
% Wejścia:
%   U_m – wektor napięć sterujących [U_mP; U_mL] (V)
%   R   – rezystancja uzwojeń (skalar) lub macierz 2x2
R = eye(2) * R;

i_m = inv(R) * U_me;  % bardziej wydajna wersja niż inv(R) * (U - E)

end

== matlab function A_Robot_2_0_m_5_V22_SI/Model Robota 2.1/Model kinematyki1/MATLAB Function ==
  data: q input; u input; dq output
function dq = kinematyka(q, u)
% Wejście:
%   q - wektor stanu [theta; x; y]
%   u - wektor sterowania [omega; v] (prędkość kątowa i liniowa)
% Wyjście:
%   dq - pochodne stanu [dtheta; dx; dy] uwzględniające ograniczenie Pfaffa
dq=[0;0;0];
% Rozpakowanie wektora stanu
theta = q(1);  % Kąt orientacji robota
x = q(2);      % Pozycja x
y = q(3);      % Pozycja y

% Macierz kinematyki G(q)
Gq = [1,  0;
      0, cos(theta);
      0, sin(theta)];

% Wstępna pochodna stanu
dq = Gq * u;

end

== matlab function A_Robot_2_0_m_5_V22_SI/MATLAB Function2 ==
  data: t input; dtheta_d output
function dtheta_d = obl_theta(t)
    % Parametry trajektorii Lissajousa
    A = 1; B = 1;
    a = 1; b = 2;

    % Pochodne położenia
    dx = A * a * cos(a * t);
    dy = B * b * cos(b * t);

    % Drugie pochodne (przyspieszenia)
    ddx = -A * a^2 * sin(a * t);
    ddy = -B * b^2 * sin(b * t);

    % Obliczenie pochodnej kąta theta_d
    dtheta_d = (ddy * dx - ddx * dy) / (dx^2 + dy^2);
end
